simulink model "fcc"  (R2020b)
settings: Solver=VariableStepAuto  StartTime=0.0  StopTime=600  RelTol=1e-3
undefined symbols (not defined in the file): a0, a1, a2, b0, b1, b2, d, numarator, numitor
settings Model: Creator=danes  LastModifiedBy=danes

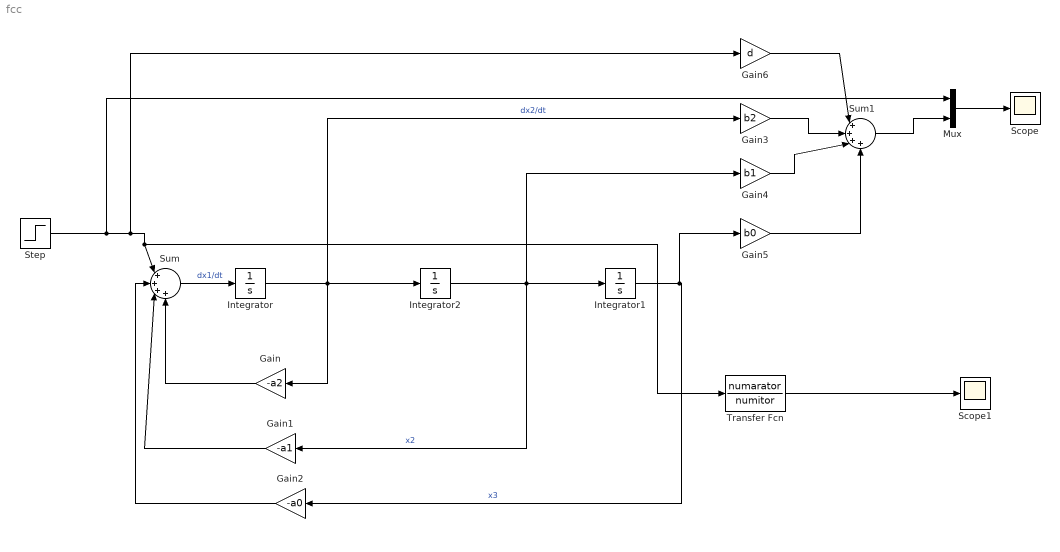
== system fcc ==
  Gain : Gain  Gain=-a2
  Gain1 : Gain  Gain=-a1
  Gain2 : Gain  Gain=-a0
  Gain3 : Gain  Gain=b2
  Gain4 : Gain  Gain=b1
  Gain5 : Gain  Gain=b0
  Gain6 : Gain  Gain=d
  Integrator : Integrator
  Integrator1 : Integrator
  Integrator2 : Integrator
  Mux : Mux  Inputs=2
  Scope : Scope
  Scope1 : Scope
  Step : Step  SampleTime=0
  Sum : Sum  Inputs=|++++
  Sum1 : Sum  Inputs=|++++
  Transfer Fcn : TransferFcn  Numerator=numarator  Denominator=numitor
  wires:
  Integrator2/1 -> Gain4/1, Gain1/1, Integrator1/1  "x2"
  Integrator/1 -> Gain3/1, Integrator2/1, Gain/1  "dx2/dt"
  Sum/1 -> Integrator/1  "dx1/dt"
  Integrator1/1 -> Gain5/1, Gain2/1  "x3"
  Gain/1 -> Sum/4
  Gain1/1 -> Sum/3
  Gain2/1 -> Sum/2
  Step/1 -> Mux/1, Transfer Fcn/1, Sum/1, Gain6/1
  Gain6/1 -> Sum1/1
  Gain3/1 -> Sum1/2
  Gain4/1 -> Sum1/3
  Gain5/1 -> Sum1/4
  Transfer Fcn/1 -> Scope1/1
  Sum1/1 -> Mux/2
  Mux/1 -> Scope/1
